simulink model "linearModel"  (R2014b)
settings: Solver=ode4  StartTime=0.0  StopTime=TIME_SIM  FixedStep=STEP_SIZE  RelTol=1e-3
values from neighbouring files (symbols this model uses):
  Bl0 = 14.54    [main.m]    (also in mainbis.m)
  k0 = 6259.3    [main.m]    (also in mainbis.m)
  Le0 = 5.65*10^(-3)    (= 0.00565)    [main.m]    (also in mainbis.m)
  mt = 52.08*10^(-3)    (= 0.05208)    [main.m]    (also in mainbis.m)
  Re = 7.9    [main.m]    (also in mainbis.m)
  Rm = 2.628    [main.m]    (also in mainbis.m)
settings Model: Creator=Kate  LastModifiedBy=Kate
settings DataIOCC: SaveState=on

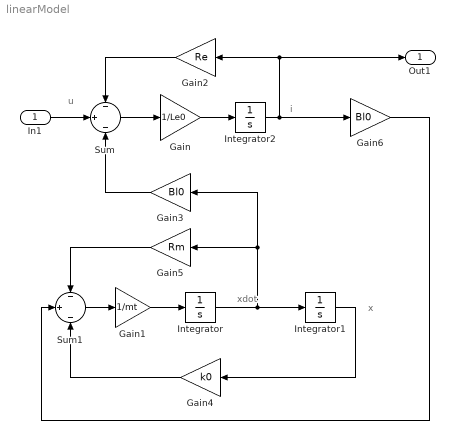
== system linearModel ==
  note: u
  note: i
  note: x
  note: xdot
  In1 : Inport
  Gain : Gain  Gain=1/Le0
  Gain1 : Gain  Gain=1/mt
  Gain2 : Gain  Gain=Re
  Gain3 : Gain  Gain=Bl0
  Gain4 : Gain  Gain=k0
  Gain5 : Gain  Gain=Rm
  Gain6 : Gain  Gain=Bl0
  Integrator : Integrator  Priority=2
  Integrator1 : Integrator  Priority=1
  Integrator2 : Integrator  Priority=3
  Sum : Sum  Inputs=-|+|-
  Sum1 : Sum  Inputs=-|+|-
  Out1 : Outport
  wires:
  Integrator/1 -> Gain3/1, Gain5/1, Integrator1/1
  Gain1/1 -> Integrator/1
  Sum1/1 -> Gain1/1
  Sum/1 -> Gain/1
  Gain/1 -> Integrator2/1
  In1/1 -> Sum/2
  Integrator2/1 -> Gain2/1, Out1/1, Gain6/1
  Gain2/1 -> Sum/1
  Integrator1/1 -> Gain4/1
  Gain3/1 -> Sum/3
  Gain4/1 -> Sum1/3
  Gain5/1 -> Sum1/1
  Gain6/1 -> Sum1/2
